simulink model "parallel_linearized"  (Simulink 7.4)
settings: Solver=ode45  StartTime=0.0  StopTime=100  FixedStep=0.05  MaxStep=0.05  RelTol=1e-3
values from neighbouring files (symbols this model uses):
  P_D = 1.08    [MpcSetup.m]    (also in get_tank_deriv.m = x(2*xsize+1); test_linearization.m = P_D_init + delta_x(end,i); test_predictions.m = 1.12)
  Ts = 0.05    [test_linearization.m]    (also in test_observer.m; test_predictions.m)
libraries: lib_compressor x2, dspsrcs4 x1
settings Model: Creator=chkajon  LastModifiedBy=chkajon
settings SFSimCC: SimUserSources=../call_qpoases_m/call_qpoases.c
settings SFSimCC: SimUserIncludeDirs=|
  | ../call_qpoases_m/qpoases3/src
  | ../call_qpoases_m/qpoases3/include

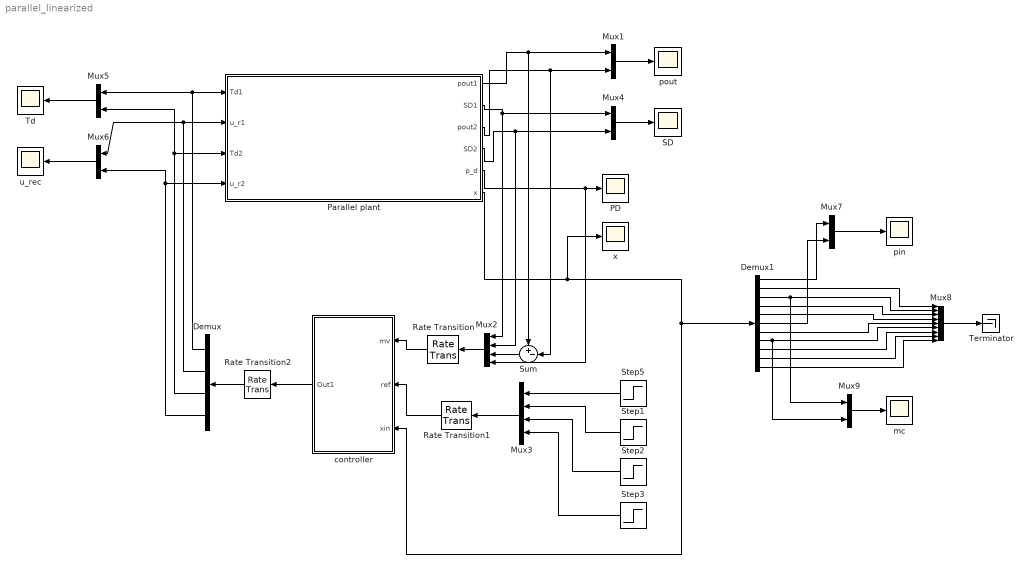
== system parallel_linearized ==
  Demux : Demux
  Demux1 : Demux  Outputs=11
  Mux{1,4..7,9} (6 alike) : Mux  Inputs=2
  Mux2 : Mux
  Mux3 : Mux
  Mux8 : Mux  Inputs=9
  PD : Scope
      settings: TimeRange=100  YMin=1.04  YMax=1.15  SaveName=SD1  DataFormat=Array
  Parallel plant : Subsystem
  Rate Transition : RateTransition  X0=[0.2;0.2;0;1.08]
  Rate Transition1 : RateTransition
  Rate Transition2 : RateTransition
  SD : Scope
      settings: TimeRange=100  YMin=-3.5  YMax=1.25  SaveName=SD3  DataFormat=Array
  Step1 : Step  Time=0  Before=0.2  After=0.2  SampleTime=0
  Step2 : Step  Time=0  After=0  SampleTime=0
  Step3 : Step  Time=0  Before=1.08  After=1.08  SampleTime=0
  Step5 : Step  Time=0  Before=0.2  After=0.2  SampleTime=0
  Sum : Sum  Inputs=+-|  OutDataType=fixdt(1, 16)  OutScaling=2^0
  Td : Scope
      settings: TimeRange=100  YMin=-0.15  YMax=0.325  SaveName=SD4  DataFormat=Array
  Terminator : Terminator
  controller : Subsystem  SystemSampleTime=Ts
  mc : Scope
      settings: TimeRange=200  YMin=0.1175  YMax=0.155  SaveName=SD8  DataFormat=Array
  pin : Scope
      settings: TimeRange=200  YMin=0.89  YMax=1  SaveName=SD7  DataFormat=Array
  pout : Scope
      settings: TimeRange=100  YMin=-0.07  YMax=0.08  SaveName=SD2  DataFormat=Array
  u_rec : Scope
      settings: TimeRange=100  YMin=-0.005  YMax=0.05  SaveName=SD5  DataFormat=Array
  x : Scope
      settings: TimeRange=85  YMin=1.1125  YMax=1.1141  SaveName=SD6  DataFormat=Array
  wires:
  controller/1(Out1) -> Rate Transition2/1
  Mux2/1 -> Rate Transition/1
  Mux3/1 -> Rate Transition1/1
  Rate Transition/1 -> controller/1(mv)
  Rate Transition1/1 -> controller/2(ref)
  Rate Transition2/1 -> Demux/1
  Demux/1 -> Parallel plant/1(Td1), Mux5/1
  Demux/2 -> Parallel plant/2(u_r1), Mux6/1
  Demux/3 -> Parallel plant/3(Td2), Mux5/2
  Demux/4 -> Parallel plant/4(u_r2), Mux6/2
  Step5/1 -> Mux3/1
  Step1/1 -> Mux3/2
  Step2/1 -> Mux3/3
  Step3/1 -> Mux3/4
  Parallel plant/1(pout1) -> Mux1/1, Sum/1
  Parallel plant/5(p_d) -> PD/1, Mux2/4
  Parallel plant/2(SD1) -> Mux4/1, Mux2/1
  Parallel plant/3(pout2) -> Mux1/2, Sum/2
  Parallel plant/4(SD2) -> Mux4/2, Mux2/2
  Mux4/1 -> SD/1
  Mux1/1 -> pout/1
  Mux5/1 -> Td/1
  Mux6/1 -> u_rec/1
  Parallel plant/6(x) -> x/1, controller/3(xin), Demux1/1
  Demux1/1 -> Mux7/1
  Demux1/6 -> Mux7/2
  Demux1/2 -> Mux8/1
  Demux1/3 -> Mux8/2, Mux9/1
  Demux1/4 -> Mux8/3
  Demux1/5 -> Mux8/4
  Demux1/7 -> Mux8/5
  Demux1/8 -> Mux8/6, Mux9/2
  Demux1/9 -> Mux8/7
  Demux1/10 -> Mux8/8
  Demux1/11 -> Mux8/9
  Mux8/1 -> Terminator/1
  Mux7/1 -> pin/1
  Mux9/1 -> mc/1
  Sum/1 -> Mux2/3

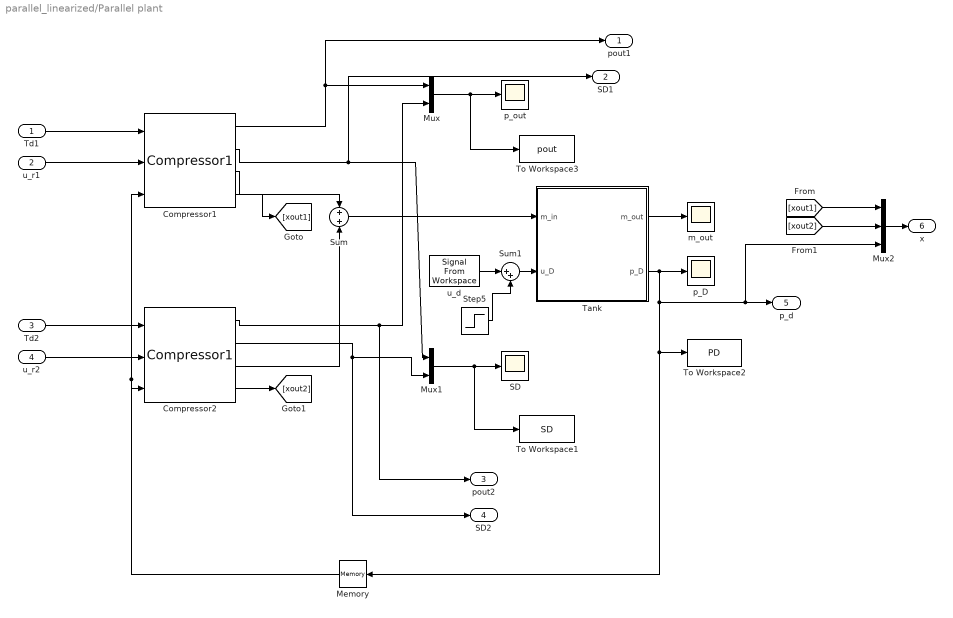
== system parallel_linearized/Parallel plant ==
  Td1 : Inport  OutDataType=fixdt(1, 16)  OutScaling=2^0
  u_r1 : Inport  Port=2  OutDataType=fixdt(1, 16)  OutScaling=2^0
  Td2 : Inport  Port=3  OutDataType=fixdt(1, 16)  OutScaling=2^0
  u_r2 : Inport  Port=4  OutDataType=fixdt(1, 16)  OutScaling=2^0
  Compressor1 : lib_compressor/Compressor1  SystemSampleTime=-1  Td_off=0.304  u_in=0.405  u_out=u_out  u_rec=0  t_delay=1  use_dist=on  u_out_dist=0  u_out_time=80  u_in_dist=-0.1  u_in_time=20
  Compressor2 : lib_compressor/Compressor1  SystemSampleTime=-1  Td_off=0.304  u_in=0.405  u_out=u_out  u_rec=0  t_delay=1  use_dist=on  u_out_dist=0  u_out_time=80  u_in_dist=-0.1  u_in_time=20
  Memory : Memory  X0=P_D
  Mux : Mux  Inputs=2
  Mux1 : Mux  Inputs=2
  Mux2 : Mux  Inputs=3
  SD : Scope
      settings: YMin=-2.5  YMax=0
  Step5 : Step  Time=50  After=0  SampleTime=0
  Sum : Sum  OutDataType=fixdt(1, 16)  OutScaling=2^0
  Sum1 : Sum  Inputs=|++  OutDataType=fixdt(1, 16)  OutScaling=2^0
  Tank : Subsystem
  To Workspace1 : ToWorkspace  VariableName=SD  SampleTime=-1  SaveFormat=Structure With Time
  To Workspace2 : ToWorkspace  VariableName=PD  SampleTime=-1  SaveFormat=Structure With Time
  To Workspace3 : ToWorkspace  VariableName=pout  SampleTime=-1  SaveFormat=Structure With Time
  m_out : Scope
      settings: SaveName=ScopeData2
  p_D : Scope
      settings: YMin=1.01  YMax=1.075  SaveName=ScopeData3
  p_out : Scope
  u_d : dspsrcs4/Signal From Workspace  SystemSampleTime=-1  X=u_d  Ts=Ts  nsamps=1  OutputAfterFinalValue=Holding final value  ignoreOrWarnInputAndFrameLengths=off
  pout1 : Outport  OutDataType=fixdt(1, 16)  OutScaling=2^0
  SD1 : Outport  Port=2  OutDataType=fixdt(1, 16)  OutScaling=2^0
  pout2 : Outport  Port=3  OutDataType=fixdt(1, 16)  OutScaling=2^0
  SD2 : Outport  Port=4  OutDataType=fixdt(1, 16)  OutScaling=2^0
  p_d : Outport  Port=5  OutDataType=fixdt(1, 16)  OutScaling=2^0
  x : Outport  Port=6  OutDataType=fixdt(1, 16)  OutScaling=2^0
  wires:
  Compressor1/3 -> Sum/1
  Tank/1(m_out) -> m_out/1
  Tank/2(p_D) -> p_D/1, To Workspace2/1, Memory/1, p_d/1, Mux2/3
  Compressor1/1 -> Mux/1, pout1/1
  Compressor1/2 -> Mux1/1, SD1/1
  Compressor2/1 -> Mux/2, pout2/1
  Compressor2/2 -> Mux1/2, SD2/1
  Td1/1 -> Compressor1/1
  u_r1/1 -> Compressor1/2
  Sum/1 -> Tank/1(m_in)
  Mux1/1 -> SD/1, To Workspace1/1
  Mux/1 -> p_out/1, To Workspace3/1
  Td2/1 -> Compressor2/1
  u_r2/1 -> Compressor2/2
  Memory/1 -> Compressor1/3, Compressor2/3
  Compressor2/3 -> Sum/2
  [xout1] -> Mux2/1
  Compressor1/4 -> [xout1]
  Compressor2/4 -> [xout2]
  [xout2] -> Mux2/2
  Mux2/1 -> x/1
  Sum1/1 -> Tank/2(u_D)
  u_d/1 -> Sum1/1
  Step5/1 -> Sum1/2

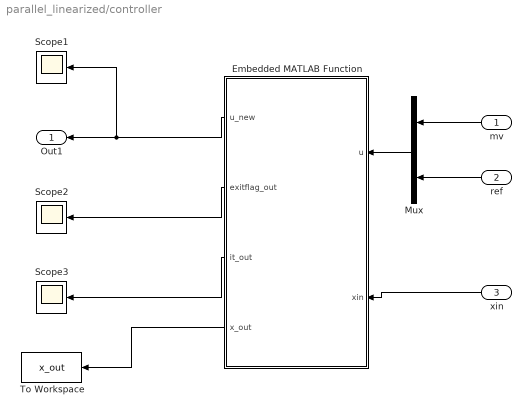
== system parallel_linearized/controller ==
  mv : Inport
  ref : Inport  Port=2
  xin : Inport  Port=3
  Embedded MATLAB Function : Stateflow chart  TreatAsAtomicUnit=on  SystemSampleTime=0.05
  Mux : Mux  Inputs=2
  Scope1 : Scope
      settings: YMin=0  YMax=0.6
  Scope2 : Scope
      settings: YMin=-1  YMax=1  SaveName=ScopeData15
  Scope3 : Scope
      settings: YMin=10  YMax=47.5  SaveName=ScopeData16
  To Workspace : ToWorkspace  VariableName=x_out  SampleTime=-1  SaveFormat=Structure With Time
  Out1 : Outport
  wires:
  mv/1 -> Mux/1
  Mux/1 -> Embedded MATLAB Function/1(u)
  ref/1 -> Mux/2
  Embedded MATLAB Function/1(u_new) -> Out1/1, Scope1/1
  Embedded MATLAB Function/3(it_out) -> Scope3/1
  Embedded MATLAB Function/2(exitflag_out) -> Scope2/1
  Embedded MATLAB Function/4(x_out) -> To Workspace/1
  xin/1 -> Embedded MATLAB Function/2(xin)

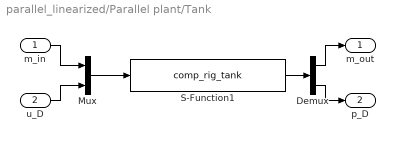
== system parallel_linearized/Parallel plant/Tank ==
  m_in : Inport  OutDataType=fixdt(1, 16)  OutScaling=2^0
  u_D : Inport  Port=2  OutDataType=fixdt(1, 16)  OutScaling=2^0
  Demux : Demux  Outputs=2
  Mux : Mux  Inputs=2
  S-Function1 : S-Function  FunctionName=comp_rig_tank  Parameters=[], P_D  EnableBusSupport=off
  m_out : Outport  OutDataType=fixdt(1, 16)  OutScaling=2^0
  p_D : Outport  Port=2  OutDataType=fixdt(1, 16)  OutScaling=2^0
  wires:
  S-Function1/1 -> Demux/1
  Demux/1 -> m_out/1
  Demux/2 -> p_D/1
  Mux/1 -> S-Function1/1
  m_in/1 -> Mux/1
  u_D/1 -> Mux/2

== matlab function controller/Embedded MATLAB Function ==
  data: u input double; u_new output double; exitflag_out output double; it_out output double; x_out output double; xin input double
function [u_new,exitflag_out,it_out,x_out]  = fcn(u,xin)
%#eml
% persistent C_new M LB UB Ga Gb Gc H Ain b A B upast xinit
persistent M LB UB Ain b upast xinit dxaug y_old C %x_init_lin
eml.extrinsic('disp');
eml.extrinsic('toc');
eml.extrinsic('tic');
eml.extrinsic('num2str');
eml.extrinsic('keyboard');
eml.extrinsic('quadprog');



[n_delay,dsize,ucontrolsize,p,m] = const_mpc();
[~, ~, xsize, ~, ysize] = const_sim();
usize=2*ucontrolsize;

if isempty(M)
    tic
    [C,M,UB,LB,b,Ain,xinit,upast] = get_constant_matrices();
    dxaug = zeros(size(xinit));
    y_old = zeros(ysize,1);
    time = toc;
    disp(['Preparation time: ' num2str(time)]);
end


y = u(1:ysize);

% Estimate state info
dxaug = dxaug + M*(y - y_old - C*(dxaug));

% Use state input info to calculate x, y
xinit(1:xsize) = xinit(1:xsize)+dxaug(1:xsize);
xinit(xsize+1:end) = dxaug(xsize+1:end);
x_out = xinit;

y_old = y;

yref = u(ysize+1:end);

% Get matrices - linearize about delayed rec.open input
[A,B,C,H,Ga,Gb,Gc,df0,Sx,Su,Sf,UWT] = get_qp_matrices(xinit,upast);



% Get reference and input vector

Yref = zeros(p*ysize,1);
Upast = zeros(m*usize,1);
for i=1:p
    Yref(1+(i-1)*ysize:i*ysize,1) = yref - y;
end
for i=1:m
    Upast(1+(i-1)*usize:i*usize,1) = upast;
end

% Update bounds
LBa = LB - Upast;
UBa = UB - Upast;

% Calculate initial state
dx0 = [zeros(xsize,1); xinit(xsize+1:xsize+n_delay(2))-upast(2); xinit(xsize+n_delay(2)+1:xsize+2*n_delay(2))-upast(4); zeros(2*dsize,1)];


% Gradient vector
f = df0'*Gc - Yref'*Ga + dx0'*Gb;% + Upast'*UWT;

% Solve QP
lbA = -inf(size(Ain,1),1);
[usol,~,exitflag,it] = call_qpoases_m(H,f,Ain,LBa,UBa,lbA,b);
exitflag_out = exitflag(1,1);
it_out = it(1,1);

if exitflag_out~=0
    exitflag_out
    usol = zeros(m*usize,1);
end


% Apply next input
delta_u = usol(1:usize,1);
u_new = upast + delta_u;


% value of x about which we linearized
xlin = dxaug;
xlin(xsize+1:end) = 0;
xlin(xsize+1) = upast(2);
xlin(xsize+1+n_delay(2)) = upast(4);

dxaug = B*[u_new(1)-upast(1);u_new(2);u_new(3)-upast(3);u_new(4)] + A*(dxaug-xlin) + df0;

upast = u_new;
